simulink model "archi"  (R2017b)
settings: Solver=FixedStepDiscrete  StartTime=0.0  StopTime=inf  RelTol=1e-3
settings Model: Creator=bourlot  LastModifiedBy=bourlot
settings SolverCC: AutoInsertRateTranBlk=on
settings DataIOCC: LimitDataPoints=on  SaveOutput=off  SignalLogging=off  DSMLogging=off  SaveTime=off
settings OptimizationCC: LifeSpan=inf
settings DebuggingCC: AlgebraicLoopMsg=error  SingleTaskRateTransMsg=error  AllowSymbolicDim=off  SFUnexpectedBacktrackingDiag=warning  SFNoUnconditionalDefaultTransitionDiag=warning  SFExecutionAtInitializationDiag=none
settings CodeAppCC: StateflowObjectComments=on
settings GRTTargetCC: TargetLangStandard=C89/C90 (ANSI)  GeneratePreprocessorConditionals=Disable all

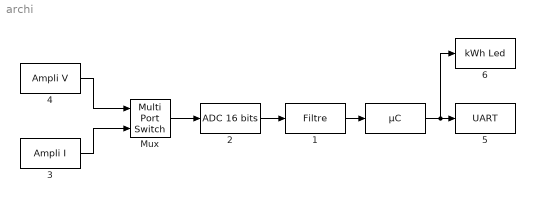
== system archi ==
  " " : Fcn  Expr=µC
  " 1" : Fcn  Expr=Filtre
  " 2" : Fcn  Expr=ADC 16 bits
  " 3" : Fcn  Expr=Ampli I
  " 4" : Fcn  Expr=Ampli V
  " 5" : Fcn  Expr=UART
  " 6" : Fcn  Expr=kWh Led
  Mux : MultiPortSwitch  DataPortOrder=Zero-based contiguous  Inputs=1  zeroidx=on
  wires:
  Mux/1 -> " 2"/1
  " 2"/1 -> " 1"/1
  " 1"/1 -> " "/1
  " 3"/1 -> Mux/2
  " 4"/1 -> Mux/1
  " "/1 -> " 6"/1, " 5"/1
